simulink model "VCO_15N_2nd_order_2020a_v2"  (R2020b)
settings: Solver=VariableStepAuto  StartTime=0.0  StopTime=5000*clk_p  RelTol=1e-3
values from neighbouring files (symbols this model uses):
  clk_p = 1/clk    (= 5e-09)    [parallel_simulink_test8.m]
  finw = 2*pi*M/(N_in*clk_p)    (= 3374757.73335)    [parallel_simulink_test8.m]
undefined symbols (not defined in the file or in its folder): Amp_in, Bias, gain_DAC
libraries: commsynccomp2 x60, simulink_extras x9, eeGeneralControl x3
(part 2 of 2)

== system VCO_15N_2nd_order_2020a_v2/15-Stage Ring Oscillator4/Convert to Square Wave1 ==
  In1 : Inport
  Constant4 : Constant  Value=0
  Relational Operator : RelationalOperator  Operator=>  RndMeth=Nearest  InputSameDT=on
  Out1 : Outport
  wires:
  Relational Operator/1 -> Out1/1
  In1/1 -> Relational Operator/1
  Constant4/1 -> Relational Operator/2

== system VCO_15N_2nd_order_2020a_v2/15-Stage Ring Oscillator4/Convert to Square Wave10 ==
  In1 : Inport
  Constant4 : Constant  Value=0
  Relational Operator : RelationalOperator  Operator=>  RndMeth=Nearest  InputSameDT=on
  Out1 : Outport
  wires:
  Relational Operator/1 -> Out1/1
  In1/1 -> Relational Operator/1
  Constant4/1 -> Relational Operator/2

== system VCO_15N_2nd_order_2020a_v2/15-Stage Ring Oscillator4/Convert to Square Wave11 ==
  In1 : Inport
  Constant4 : Constant  Value=0
  Relational Operator : RelationalOperator  Operator=>  RndMeth=Nearest  InputSameDT=on
  Out1 : Outport
  wires:
  Relational Operator/1 -> Out1/1
  In1/1 -> Relational Operator/1
  Constant4/1 -> Relational Operator/2

== system VCO_15N_2nd_order_2020a_v2/15-Stage Ring Oscillator4/Convert to Square Wave12 ==
  In1 : Inport
  Constant4 : Constant  Value=0
  Relational Operator : RelationalOperator  Operator=>  RndMeth=Nearest  InputSameDT=on
  Out1 : Outport
  wires:
  Relational Operator/1 -> Out1/1
  In1/1 -> Relational Operator/1
  Constant4/1 -> Relational Operator/2

== system VCO_15N_2nd_order_2020a_v2/15-Stage Ring Oscillator4/Convert to Square Wave14 ==
  In1 : Inport
  Constant4 : Constant  Value=0
  Relational Operator : RelationalOperator  Operator=>  RndMeth=Nearest  InputSameDT=on
  Out1 : Outport
  wires:
  Relational Operator/1 -> Out1/1
  In1/1 -> Relational Operator/1
  Constant4/1 -> Relational Operator/2

== system VCO_15N_2nd_order_2020a_v2/15-Stage Ring Oscillator4/Convert to Square Wave15 ==
  In1 : Inport
  Constant4 : Constant  Value=0
  Relational Operator : RelationalOperator  Operator=>  RndMeth=Nearest  InputSameDT=on
  Out1 : Outport
  wires:
  Relational Operator/1 -> Out1/1
  In1/1 -> Relational Operator/1
  Constant4/1 -> Relational Operator/2

== system VCO_15N_2nd_order_2020a_v2/15-Stage Ring Oscillator4/Convert to Square Wave2 ==
  In1 : Inport
  Constant4 : Constant  Value=0
  Relational Operator : RelationalOperator  Operator=>  RndMeth=Nearest  InputSameDT=on
  Out1 : Outport
  wires:
  Relational Operator/1 -> Out1/1
  In1/1 -> Relational Operator/1
  Constant4/1 -> Relational Operator/2

== system VCO_15N_2nd_order_2020a_v2/15-Stage Ring Oscillator4/Convert to Square Wave3 ==
  In1 : Inport
  Constant4 : Constant  Value=0
  Relational Operator : RelationalOperator  Operator=>  RndMeth=Nearest  InputSameDT=on
  Out1 : Outport
  wires:
  Relational Operator/1 -> Out1/1
  In1/1 -> Relational Operator/1
  Constant4/1 -> Relational Operator/2

== system VCO_15N_2nd_order_2020a_v2/15-Stage Ring Oscillator4/Convert to Square Wave4 ==
  In1 : Inport
  Constant4 : Constant  Value=0
  Relational Operator : RelationalOperator  Operator=>  RndMeth=Nearest  InputSameDT=on
  Out1 : Outport
  wires:
  Relational Operator/1 -> Out1/1
  In1/1 -> Relational Operator/1
  Constant4/1 -> Relational Operator/2

== system VCO_15N_2nd_order_2020a_v2/15-Stage Ring Oscillator4/Convert to Square Wave5 ==
  In1 : Inport
  Constant4 : Constant  Value=0
  Relational Operator : RelationalOperator  Operator=>  RndMeth=Nearest  InputSameDT=on
  Out1 : Outport
  wires:
  Relational Operator/1 -> Out1/1
  In1/1 -> Relational Operator/1
  Constant4/1 -> Relational Operator/2

== system VCO_15N_2nd_order_2020a_v2/15-Stage Ring Oscillator4/Convert to Square Wave6 ==
  In1 : Inport
  Constant4 : Constant  Value=0
  Relational Operator : RelationalOperator  Operator=>  RndMeth=Nearest  InputSameDT=on
  Out1 : Outport
  wires:
  Relational Operator/1 -> Out1/1
  In1/1 -> Relational Operator/1
  Constant4/1 -> Relational Operator/2

== system VCO_15N_2nd_order_2020a_v2/15-Stage Ring Oscillator4/Convert to Square Wave7 ==
  In1 : Inport
  Constant4 : Constant  Value=0
  Relational Operator : RelationalOperator  Operator=>  RndMeth=Nearest  InputSameDT=on
  Out1 : Outport
  wires:
  Relational Operator/1 -> Out1/1
  In1/1 -> Relational Operator/1
  Constant4/1 -> Relational Operator/2

== system VCO_15N_2nd_order_2020a_v2/15-Stage Ring Oscillator4/Convert to Square Wave8 ==
  In1 : Inport
  Constant4 : Constant  Value=0
  Relational Operator : RelationalOperator  Operator=>  RndMeth=Nearest  InputSameDT=on
  Out1 : Outport
  wires:
  Relational Operator/1 -> Out1/1
  In1/1 -> Relational Operator/1
  Constant4/1 -> Relational Operator/2

== system VCO_15N_2nd_order_2020a_v2/15-Stage Ring Oscillator4/Convert to Square Wave9 ==
  In1 : Inport
  Constant4 : Constant  Value=0
  Relational Operator : RelationalOperator  Operator=>  RndMeth=Nearest  InputSameDT=on
  Out1 : Outport
  wires:
  Relational Operator/1 -> Out1/1
  In1/1 -> Relational Operator/1
  Constant4/1 -> Relational Operator/2
